simulink model "BD_PAR_AUTO_base_model"  (Simulink 10.3)
settings: Solver=ode1  StartTime=0.0  StopTime=max(cyc_mph(:,1))  FixedStep=1  MaxStep=1  RelTol=1e-3  AbsTol=1e-3
undefined symbols (not defined in the file): acc_dcdc_eff, acc_elec_eff, acc_elec_pwr, acc_mech_eff, acc_mech_pwr, acc_mech_trq, air_cp, amb_tmp, cs_charge_deplete_bool, cs_charge_trq, cs_electric_decel_spd, cs_electric_launch_spd_hi, cs_electric_launch_spd_lo, cs_hi_soc, cs_lo_soc, cs_min_trq_frac, cs_off_trq_frac, cyc_avg_time, cyc_cargo_mass, cyc_elevation_init, cyc_filter_bool, cyc_grade, cyc_mph, enable_sim_stop_distance, enable_sim_stop_max_spd, enable_sim_stop_speed, enable_sim_stop_time, enable_stop, enable_stop_fc, ess_cap_scale, ess_coulombic_eff, ess_init_soc, ess_max_ah_cap, ess_max_volts, ess_min_volts, ess_mod_airflow, ess_mod_cp, ess_mod_init_tmp, ess_module_mass, ess_module_num, ess_on, ess_r_chg, ess_r_dis, ess_res_scale_coef, ess_res_scale_fun, ess_set_tmp, ess_soc, ess_th_calc, ess_th_res_off, ess_th_res_on, ess_tmp, ess_voc, ex_calc, ex_cat_co_frac, ex_cat_ext_cp, ex_cat_ext_emisv, ex_cat_ext_init_tmp, ex_cat_ext_mass, ex_cat_ext_sarea, ex_cat_hc_frac ... (+168)
(part 14 of 15)

== system BD_PAR_AUTO_base_model/electric acc loads <acc>/Electrical Accessory Loads v2 <acc>/backward model/electrical accessories (W)/Electrical Accessories: Time Variable/Elec Aux Loads 14V Pwr/RearHVAC/Subsystem/Subsystem1/ToggleTimes ==
  Constant : Constant  Value=ToggleTimes  VectorParams1D=off
  Out1 : Outport
  wires:
  Constant/1 -> Out1/1

== system BD_PAR_AUTO_base_model/electric acc loads <acc>/Electrical Accessory Loads v2 <acc>/backward model/electrical accessories (W)/Electrical Accessories: Time Variable/Elec Aux Loads 14V Pwr/RearHVAC/Subsystem/Subsystem1/Triggered Subsystem1 ==
  In1 : Inport
  Enable : EnablePort
  Constant1 : Constant
  Constant2 : Constant  Value=0
  Constant3 : Constant  Value=0
  Relational Operator : RelationalOperator  Operator===  RndMeth=Nearest  InputSameDT=on
  Switch : Switch  Threshold=.5
  Out1 : Outport  InitialOutput=InitialOn
  wires:
  Switch/1 -> Out1/1
  Constant3/1 -> Switch/3
  Constant1/1 -> Switch/1
  Relational Operator/1 -> Switch/2
  Constant2/1 -> Relational Operator/2
  In1/1 -> Relational Operator/1

== system BD_PAR_AUTO_base_model/electric acc loads <acc>/Electrical Accessory Loads v2 <acc>/backward model/electrical accessories (W)/Electrical Accessories: Time Variable/Elec Aux Loads 14V Pwr/RearWipers/Subsystem/Subsystem/DurationOn1 ==
  Constant : Constant  Value=DurationOn
  Out1 : Outport
  wires:
  Constant/1 -> Out1/1

== system BD_PAR_AUTO_base_model/electric acc loads <acc>/Electrical Accessory Loads v2 <acc>/backward model/electrical accessories (W)/Electrical Accessories: Time Variable/Elec Aux Loads 14V Pwr/RearWipers/Subsystem/Subsystem/Period1 ==
  Constant : Constant  Value=Period
  Out1 : Outport
  wires:
  Constant/1 -> Out1/1

== system BD_PAR_AUTO_base_model/electric acc loads <acc>/Electrical Accessory Loads v2 <acc>/backward model/electrical accessories (W)/Electrical Accessories: Time Variable/Elec Aux Loads 14V Pwr/RearWipers/Subsystem/Subsystem/StartTime1 ==
  Constant : Constant  Value=StartTime
  Out1 : Outport
  wires:
  Constant/1 -> Out1/1

== system BD_PAR_AUTO_base_model/electric acc loads <acc>/Electrical Accessory Loads v2 <acc>/backward model/electrical accessories (W)/Electrical Accessories: Time Variable/Elec Aux Loads 14V Pwr/RearWipers/Subsystem/Subsystem/StartTime3 ==
  Constant : Constant  Value=StartTime
  Out1 : Outport
  wires:
  Constant/1 -> Out1/1

== system BD_PAR_AUTO_base_model/electric acc loads <acc>/Electrical Accessory Loads v2 <acc>/backward model/electrical accessories (W)/Electrical Accessories: Time Variable/Elec Aux Loads 14V Pwr/RearWipers/Subsystem/Subsystem/Triggered Subsystem2 ==
  time : Inport
  Trigger : TriggerPort  VariantControl=(inherit)
  last trig on time : Outport  InitialOutput=StartTime
  wires:
  time/1 -> last trig on time/1

== system BD_PAR_AUTO_base_model/electric acc loads <acc>/Electrical Accessory Loads v2 <acc>/backward model/electrical accessories (W)/Electrical Accessories: Time Variable/Elec Aux Loads 14V Pwr/RearWipers/Subsystem/Subsystem1/ToggleTimes ==
  Constant : Constant  Value=ToggleTimes  VectorParams1D=off
  Out1 : Outport
  wires:
  Constant/1 -> Out1/1

== system BD_PAR_AUTO_base_model/electric acc loads <acc>/Electrical Accessory Loads v2 <acc>/backward model/electrical accessories (W)/Electrical Accessories: Time Variable/Elec Aux Loads 14V Pwr/RearWipers/Subsystem/Subsystem1/Triggered Subsystem1 ==
  In1 : Inport
  Enable : EnablePort
  Constant1 : Constant
  Constant2 : Constant  Value=0
  Constant3 : Constant  Value=0
  Relational Operator : RelationalOperator  Operator===  RndMeth=Nearest  InputSameDT=on
  Switch : Switch  Threshold=.5
  Out1 : Outport  InitialOutput=InitialOn
  wires:
  Switch/1 -> Out1/1
  Constant3/1 -> Switch/3
  Constant1/1 -> Switch/1
  Relational Operator/1 -> Switch/2
  Constant2/1 -> Relational Operator/2
  In1/1 -> Relational Operator/1

== system BD_PAR_AUTO_base_model/electric acc loads <acc>/Electrical Accessory Loads v2 <acc>/backward model/electrical accessories (W)/Electrical Accessories: Time Variable/Elec Aux Loads 14V Pwr/Starter/Starter/Subsystem/Last Engine On Time ==
  In1 : Inport
  Trigger : TriggerPort  VariantControl=(inherit)
  Out1 : Outport  InitialOutput=-100
  wires:
  In1/1 -> Out1/1

== system BD_PAR_AUTO_base_model/electric acc loads <acc>/Electrical Accessory Loads v2 <acc>/backward model/electrical accessories (W)/Electrical Accessories: Time Variable/Elec Aux Loads 14V Pwr/TurnSignals/Subsystem/Subsystem/DurationOn1 ==
  Constant : Constant  Value=DurationOn
  Out1 : Outport
  wires:
  Constant/1 -> Out1/1

== system BD_PAR_AUTO_base_model/electric acc loads <acc>/Electrical Accessory Loads v2 <acc>/backward model/electrical accessories (W)/Electrical Accessories: Time Variable/Elec Aux Loads 14V Pwr/TurnSignals/Subsystem/Subsystem/Period1 ==
  Constant : Constant  Value=Period
  Out1 : Outport
  wires:
  Constant/1 -> Out1/1

== system BD_PAR_AUTO_base_model/electric acc loads <acc>/Electrical Accessory Loads v2 <acc>/backward model/electrical accessories (W)/Electrical Accessories: Time Variable/Elec Aux Loads 14V Pwr/TurnSignals/Subsystem/Subsystem/StartTime1 ==
  Constant : Constant  Value=StartTime
  Out1 : Outport
  wires:
  Constant/1 -> Out1/1

== system BD_PAR_AUTO_base_model/electric acc loads <acc>/Electrical Accessory Loads v2 <acc>/backward model/electrical accessories (W)/Electrical Accessories: Time Variable/Elec Aux Loads 14V Pwr/TurnSignals/Subsystem/Subsystem/StartTime3 ==
  Constant : Constant  Value=StartTime
  Out1 : Outport
  wires:
  Constant/1 -> Out1/1

== system BD_PAR_AUTO_base_model/electric acc loads <acc>/Electrical Accessory Loads v2 <acc>/backward model/electrical accessories (W)/Electrical Accessories: Time Variable/Elec Aux Loads 14V Pwr/TurnSignals/Subsystem/Subsystem/Triggered Subsystem2 ==
  time : Inport
  Trigger : TriggerPort  VariantControl=(inherit)
  last trig on time : Outport  InitialOutput=StartTime
  wires:
  time/1 -> last trig on time/1

== system BD_PAR_AUTO_base_model/electric acc loads <acc>/Electrical Accessory Loads v2 <acc>/backward model/electrical accessories (W)/Electrical Accessories: Time Variable/Elec Aux Loads 14V Pwr/TurnSignals/Subsystem/Subsystem1/ToggleTimes ==
  Constant : Constant  Value=ToggleTimes  VectorParams1D=off
  Out1 : Outport
  wires:
  Constant/1 -> Out1/1

== system BD_PAR_AUTO_base_model/electric acc loads <acc>/Electrical Accessory Loads v2 <acc>/backward model/electrical accessories (W)/Electrical Accessories: Time Variable/Elec Aux Loads 14V Pwr/TurnSignals/Subsystem/Subsystem1/Triggered Subsystem1 ==
  In1 : Inport
  Enable : EnablePort
  Constant1 : Constant
  Constant2 : Constant  Value=0
  Constant3 : Constant  Value=0
  Relational Operator : RelationalOperator  Operator===  RndMeth=Nearest  InputSameDT=on
  Switch : Switch  Threshold=.5
  Out1 : Outport  InitialOutput=InitialOn
  wires:
  Switch/1 -> Out1/1
  Constant3/1 -> Switch/3
  Constant1/1 -> Switch/1
  Relational Operator/1 -> Switch/2
  Constant2/1 -> Relational Operator/2
  In1/1 -> Relational Operator/1

== system BD_PAR_AUTO_base_model/electric acc loads <acc>/Electrical Accessory Loads v2 <acc>/backward model/electrical accessories (W)/Electrical Accessories: Time Variable/Elec Aux Loads HiV Pwr/CurrentLoad1/Subsystem/Subsystem/DurationOn1 ==
  Constant : Constant  Value=DurationOn
  Out1 : Outport
  wires:
  Constant/1 -> Out1/1

== system BD_PAR_AUTO_base_model/electric acc loads <acc>/Electrical Accessory Loads v2 <acc>/backward model/electrical accessories (W)/Electrical Accessories: Time Variable/Elec Aux Loads HiV Pwr/CurrentLoad1/Subsystem/Subsystem/Period1 ==
  Constant : Constant  Value=Period
  Out1 : Outport
  wires:
  Constant/1 -> Out1/1

== system BD_PAR_AUTO_base_model/electric acc loads <acc>/Electrical Accessory Loads v2 <acc>/backward model/electrical accessories (W)/Electrical Accessories: Time Variable/Elec Aux Loads HiV Pwr/CurrentLoad1/Subsystem/Subsystem/StartTime1 ==
  Constant : Constant  Value=StartTime
  Out1 : Outport
  wires:
  Constant/1 -> Out1/1

== system BD_PAR_AUTO_base_model/electric acc loads <acc>/Electrical Accessory Loads v2 <acc>/backward model/electrical accessories (W)/Electrical Accessories: Time Variable/Elec Aux Loads HiV Pwr/CurrentLoad1/Subsystem/Subsystem/StartTime3 ==
  Constant : Constant  Value=StartTime
  Out1 : Outport
  wires:
  Constant/1 -> Out1/1

== system BD_PAR_AUTO_base_model/electric acc loads <acc>/Electrical Accessory Loads v2 <acc>/backward model/electrical accessories (W)/Electrical Accessories: Time Variable/Elec Aux Loads HiV Pwr/CurrentLoad1/Subsystem/Subsystem/Triggered Subsystem2 ==
  time : Inport
  Trigger : TriggerPort  VariantControl=(inherit)
  last trig on time : Outport  InitialOutput=StartTime
  wires:
  time/1 -> last trig on time/1

== system BD_PAR_AUTO_base_model/electric acc loads <acc>/Electrical Accessory Loads v2 <acc>/backward model/electrical accessories (W)/Electrical Accessories: Time Variable/Elec Aux Loads HiV Pwr/CurrentLoad1/Subsystem/Subsystem1/ToggleTimes ==
  Constant : Constant  Value=ToggleTimes  VectorParams1D=off
  Out1 : Outport
  wires:
  Constant/1 -> Out1/1

== system BD_PAR_AUTO_base_model/electric acc loads <acc>/Electrical Accessory Loads v2 <acc>/backward model/electrical accessories (W)/Electrical Accessories: Time Variable/Elec Aux Loads HiV Pwr/CurrentLoad1/Subsystem/Subsystem1/Triggered Subsystem1 ==
  In1 : Inport
  Enable : EnablePort
  Constant1 : Constant
  Constant2 : Constant  Value=0
  Constant3 : Constant  Value=0
  Relational Operator : RelationalOperator  Operator===  RndMeth=Nearest  InputSameDT=on
  Switch : Switch  Threshold=.5
  Out1 : Outport  InitialOutput=InitialOn
  wires:
  Switch/1 -> Out1/1
  Constant3/1 -> Switch/3
  Constant1/1 -> Switch/1
  Relational Operator/1 -> Switch/2
  Constant2/1 -> Relational Operator/2
  In1/1 -> Relational Operator/1

== system BD_PAR_AUTO_base_model/electric acc loads <acc>/Electrical Accessory Loads v2 <acc>/backward model/electrical accessories (W)/Electrical Accessories: Time Variable/Elec Aux Loads HiV Pwr/PowerLoad1/Subsystem/Subsystem/DurationOn1 ==
  Constant : Constant  Value=DurationOn
  Out1 : Outport
  wires:
  Constant/1 -> Out1/1

== system BD_PAR_AUTO_base_model/electric acc loads <acc>/Electrical Accessory Loads v2 <acc>/backward model/electrical accessories (W)/Electrical Accessories: Time Variable/Elec Aux Loads HiV Pwr/PowerLoad1/Subsystem/Subsystem/Period1 ==
  Constant : Constant  Value=Period
  Out1 : Outport
  wires:
  Constant/1 -> Out1/1

== system BD_PAR_AUTO_base_model/electric acc loads <acc>/Electrical Accessory Loads v2 <acc>/backward model/electrical accessories (W)/Electrical Accessories: Time Variable/Elec Aux Loads HiV Pwr/PowerLoad1/Subsystem/Subsystem/StartTime1 ==
  Constant : Constant  Value=StartTime
  Out1 : Outport
  wires:
  Constant/1 -> Out1/1

== system BD_PAR_AUTO_base_model/electric acc loads <acc>/Electrical Accessory Loads v2 <acc>/backward model/electrical accessories (W)/Electrical Accessories: Time Variable/Elec Aux Loads HiV Pwr/PowerLoad1/Subsystem/Subsystem/StartTime3 ==
  Constant : Constant  Value=StartTime
  Out1 : Outport
  wires:
  Constant/1 -> Out1/1

== system BD_PAR_AUTO_base_model/electric acc loads <acc>/Electrical Accessory Loads v2 <acc>/backward model/electrical accessories (W)/Electrical Accessories: Time Variable/Elec Aux Loads HiV Pwr/PowerLoad1/Subsystem/Subsystem/Triggered Subsystem2 ==
  time : Inport
  Trigger : TriggerPort  VariantControl=(inherit)
  last trig on time : Outport  InitialOutput=StartTime
  wires:
  time/1 -> last trig on time/1

== system BD_PAR_AUTO_base_model/electric acc loads <acc>/Electrical Accessory Loads v2 <acc>/backward model/electrical accessories (W)/Electrical Accessories: Time Variable/Elec Aux Loads HiV Pwr/PowerLoad1/Subsystem/Subsystem1/ToggleTimes ==
  Constant : Constant  Value=ToggleTimes  VectorParams1D=off
  Out1 : Outport
  wires:
  Constant/1 -> Out1/1

== system BD_PAR_AUTO_base_model/electric acc loads <acc>/Electrical Accessory Loads v2 <acc>/backward model/electrical accessories (W)/Electrical Accessories: Time Variable/Elec Aux Loads HiV Pwr/PowerLoad1/Subsystem/Subsystem1/Triggered Subsystem1 ==
  In1 : Inport
  Enable : EnablePort
  Constant1 : Constant
  Constant2 : Constant  Value=0
  Constant3 : Constant  Value=0
  Relational Operator : RelationalOperator  Operator===  RndMeth=Nearest  InputSameDT=on
  Switch : Switch  Threshold=.5
  Out1 : Outport  InitialOutput=InitialOn
  wires:
  Switch/1 -> Out1/1
  Constant3/1 -> Switch/3
  Constant1/1 -> Switch/1
  Relational Operator/1 -> Switch/2
  Constant2/1 -> Relational Operator/2
  In1/1 -> Relational Operator/1

== system BD_PAR_AUTO_base_model/electric acc loads <acc>/Electrical Accessory Loads v2 <acc>/backward model/electrical accessories (W)/Electrical Accessories: Time Variable/Elec Aux Loads HiV Pwr/PowerLoad2/Subsystem/Subsystem/DurationOn1 ==
  Constant : Constant  Value=DurationOn
  Out1 : Outport
  wires:
  Constant/1 -> Out1/1

== system BD_PAR_AUTO_base_model/electric acc loads <acc>/Electrical Accessory Loads v2 <acc>/backward model/electrical accessories (W)/Electrical Accessories: Time Variable/Elec Aux Loads HiV Pwr/PowerLoad2/Subsystem/Subsystem/Period1 ==
  Constant : Constant  Value=Period
  Out1 : Outport
  wires:
  Constant/1 -> Out1/1

== system BD_PAR_AUTO_base_model/electric acc loads <acc>/Electrical Accessory Loads v2 <acc>/backward model/electrical accessories (W)/Electrical Accessories: Time Variable/Elec Aux Loads HiV Pwr/PowerLoad2/Subsystem/Subsystem/StartTime1 ==
  Constant : Constant  Value=StartTime
  Out1 : Outport
  wires:
  Constant/1 -> Out1/1

== system BD_PAR_AUTO_base_model/electric acc loads <acc>/Electrical Accessory Loads v2 <acc>/backward model/electrical accessories (W)/Electrical Accessories: Time Variable/Elec Aux Loads HiV Pwr/PowerLoad2/Subsystem/Subsystem/StartTime3 ==
  Constant : Constant  Value=StartTime
  Out1 : Outport
  wires:
  Constant/1 -> Out1/1

== system BD_PAR_AUTO_base_model/electric acc loads <acc>/Electrical Accessory Loads v2 <acc>/backward model/electrical accessories (W)/Electrical Accessories: Time Variable/Elec Aux Loads HiV Pwr/PowerLoad2/Subsystem/Subsystem/Triggered Subsystem2 ==
  time : Inport
  Trigger : TriggerPort  VariantControl=(inherit)
  last trig on time : Outport  InitialOutput=StartTime
  wires:
  time/1 -> last trig on time/1

== system BD_PAR_AUTO_base_model/electric acc loads <acc>/Electrical Accessory Loads v2 <acc>/backward model/electrical accessories (W)/Electrical Accessories: Time Variable/Elec Aux Loads HiV Pwr/PowerLoad2/Subsystem/Subsystem1/ToggleTimes ==
  Constant : Constant  Value=ToggleTimes  VectorParams1D=off
  Out1 : Outport
  wires:
  Constant/1 -> Out1/1

== system BD_PAR_AUTO_base_model/electric acc loads <acc>/Electrical Accessory Loads v2 <acc>/backward model/electrical accessories (W)/Electrical Accessories: Time Variable/Elec Aux Loads HiV Pwr/PowerLoad2/Subsystem/Subsystem1/Triggered Subsystem1 ==
  In1 : Inport
  Enable : EnablePort
  Constant1 : Constant
  Constant2 : Constant  Value=0
  Constant3 : Constant  Value=0
  Relational Operator : RelationalOperator  Operator===  RndMeth=Nearest  InputSameDT=on
  Switch : Switch  Threshold=.5
  Out1 : Outport  InitialOutput=InitialOn
  wires:
  Switch/1 -> Out1/1
  Constant3/1 -> Switch/3
  Constant1/1 -> Switch/1
  Relational Operator/1 -> Switch/2
  Constant2/1 -> Relational Operator/2
  In1/1 -> Relational Operator/1

== system BD_PAR_AUTO_base_model/electric acc loads <acc>/Electrical Accessory Loads v2 <acc>/backward model/electrical accessories (W)/Electrical Accessories: Time Variable/Elec Aux Loads HiV Pwr/PowerLoad3/Subsystem/Subsystem/DurationOn1 ==
  Constant : Constant  Value=DurationOn
  Out1 : Outport
  wires:
  Constant/1 -> Out1/1

== system BD_PAR_AUTO_base_model/electric acc loads <acc>/Electrical Accessory Loads v2 <acc>/backward model/electrical accessories (W)/Electrical Accessories: Time Variable/Elec Aux Loads HiV Pwr/PowerLoad3/Subsystem/Subsystem/Period1 ==
  Constant : Constant  Value=Period
  Out1 : Outport
  wires:
  Constant/1 -> Out1/1

== system BD_PAR_AUTO_base_model/electric acc loads <acc>/Electrical Accessory Loads v2 <acc>/backward model/electrical accessories (W)/Electrical Accessories: Time Variable/Elec Aux Loads HiV Pwr/PowerLoad3/Subsystem/Subsystem/StartTime1 ==
  Constant : Constant  Value=StartTime
  Out1 : Outport
  wires:
  Constant/1 -> Out1/1

== system BD_PAR_AUTO_base_model/electric acc loads <acc>/Electrical Accessory Loads v2 <acc>/backward model/electrical accessories (W)/Electrical Accessories: Time Variable/Elec Aux Loads HiV Pwr/PowerLoad3/Subsystem/Subsystem/StartTime3 ==
  Constant : Constant  Value=StartTime
  Out1 : Outport
  wires:
  Constant/1 -> Out1/1

== system BD_PAR_AUTO_base_model/electric acc loads <acc>/Electrical Accessory Loads v2 <acc>/backward model/electrical accessories (W)/Electrical Accessories: Time Variable/Elec Aux Loads HiV Pwr/PowerLoad3/Subsystem/Subsystem/Triggered Subsystem2 ==
  time : Inport
  Trigger : TriggerPort  VariantControl=(inherit)
  last trig on time : Outport  InitialOutput=StartTime
  wires:
  time/1 -> last trig on time/1

== system BD_PAR_AUTO_base_model/electric acc loads <acc>/Electrical Accessory Loads v2 <acc>/backward model/electrical accessories (W)/Electrical Accessories: Time Variable/Elec Aux Loads HiV Pwr/PowerLoad3/Subsystem/Subsystem1/ToggleTimes ==
  Constant : Constant  Value=ToggleTimes  VectorParams1D=off
  Out1 : Outport
  wires:
  Constant/1 -> Out1/1

== system BD_PAR_AUTO_base_model/electric acc loads <acc>/Electrical Accessory Loads v2 <acc>/backward model/electrical accessories (W)/Electrical Accessories: Time Variable/Elec Aux Loads HiV Pwr/PowerLoad3/Subsystem/Subsystem1/Triggered Subsystem1 ==
  In1 : Inport
  Enable : EnablePort
  Constant1 : Constant
  Constant2 : Constant  Value=0
  Constant3 : Constant  Value=0
  Relational Operator : RelationalOperator  Operator===  RndMeth=Nearest  InputSameDT=on
  Switch : Switch  Threshold=.5
  Out1 : Outport  InitialOutput=InitialOn
  wires:
  Switch/1 -> Out1/1
  Constant3/1 -> Switch/3
  Constant1/1 -> Switch/1
  Relational Operator/1 -> Switch/2
  Constant2/1 -> Relational Operator/2
  In1/1 -> Relational Operator/1

== system BD_PAR_AUTO_base_model/electric acc loads <acc>/Electrical Accessory Loads v2 <acc>/backward model/electrical accessories (W)/Electrical Accessories: Time Variable/Elec Aux Loads HiV Pwr/SpeedLoad1/Subsystem/Subsystem/DurationOn1 ==
  Constant : Constant  Value=DurationOn
  Out1 : Outport
  wires:
  Constant/1 -> Out1/1

== system BD_PAR_AUTO_base_model/electric acc loads <acc>/Electrical Accessory Loads v2 <acc>/backward model/electrical accessories (W)/Electrical Accessories: Time Variable/Elec Aux Loads HiV Pwr/SpeedLoad1/Subsystem/Subsystem/Period1 ==
  Constant : Constant  Value=Period
  Out1 : Outport
  wires:
  Constant/1 -> Out1/1

== system BD_PAR_AUTO_base_model/electric acc loads <acc>/Electrical Accessory Loads v2 <acc>/backward model/electrical accessories (W)/Electrical Accessories: Time Variable/Elec Aux Loads HiV Pwr/SpeedLoad1/Subsystem/Subsystem/StartTime1 ==
  Constant : Constant  Value=StartTime
  Out1 : Outport
  wires:
  Constant/1 -> Out1/1

== system BD_PAR_AUTO_base_model/electric acc loads <acc>/Electrical Accessory Loads v2 <acc>/backward model/electrical accessories (W)/Electrical Accessories: Time Variable/Elec Aux Loads HiV Pwr/SpeedLoad1/Subsystem/Subsystem/StartTime3 ==
  Constant : Constant  Value=StartTime
  Out1 : Outport
  wires:
  Constant/1 -> Out1/1

== system BD_PAR_AUTO_base_model/electric acc loads <acc>/Electrical Accessory Loads v2 <acc>/backward model/electrical accessories (W)/Electrical Accessories: Time Variable/Elec Aux Loads HiV Pwr/SpeedLoad1/Subsystem/Subsystem/Triggered Subsystem2 ==
  time : Inport
  Trigger : TriggerPort  VariantControl=(inherit)
  last trig on time : Outport  InitialOutput=StartTime
  wires:
  time/1 -> last trig on time/1

== system BD_PAR_AUTO_base_model/electric acc loads <acc>/Electrical Accessory Loads v2 <acc>/backward model/electrical accessories (W)/Electrical Accessories: Time Variable/Elec Aux Loads HiV Pwr/SpeedLoad1/Subsystem/Subsystem1/ToggleTimes ==
  Constant : Constant  Value=ToggleTimes  VectorParams1D=off
  Out1 : Outport
  wires:
  Constant/1 -> Out1/1

== system BD_PAR_AUTO_base_model/electric acc loads <acc>/Electrical Accessory Loads v2 <acc>/backward model/electrical accessories (W)/Electrical Accessories: Time Variable/Elec Aux Loads HiV Pwr/SpeedLoad1/Subsystem/Subsystem1/Triggered Subsystem1 ==
  In1 : Inport
  Enable : EnablePort
  Constant1 : Constant
  Constant2 : Constant  Value=0
  Constant3 : Constant  Value=0
  Relational Operator : RelationalOperator  Operator===  RndMeth=Nearest  InputSameDT=on
  Switch : Switch  Threshold=.5
  Out1 : Outport  InitialOutput=InitialOn
  wires:
  Switch/1 -> Out1/1
  Constant3/1 -> Switch/3
  Constant1/1 -> Switch/1
  Relational Operator/1 -> Switch/2
  Constant2/1 -> Relational Operator/2
  In1/1 -> Relational Operator/1

== system BD_PAR_AUTO_base_model/electric acc loads <acc>/Electrical Accessory Loads v2 <acc>/backward model/electrical accessories (W)/Electrical Accessories: Time Variable/Elec Aux Loads HiV Pwr/Starter/Starter/Subsystem/Last Engine On Time ==
  In1 : Inport
  Trigger : TriggerPort  VariantControl=(inherit)
  Out1 : Outport  InitialOutput=-100
  wires:
  In1/1 -> Out1/1

== system BD_PAR_AUTO_base_model/mechanical accessory loads <acc>/Mechanical Accessory Loads v2 <acc>/backward model/mechanical accessories (Nm)/Mechanical Accessories: Const Mech Var Elect/Elec Aux Loads 14V Pwr/ExternalLights/Subsystem/Subsystem/DurationOn1 ==
  Constant : Constant  Value=DurationOn
  Out1 : Outport
  wires:
  Constant/1 -> Out1/1

== system BD_PAR_AUTO_base_model/mechanical accessory loads <acc>/Mechanical Accessory Loads v2 <acc>/backward model/mechanical accessories (Nm)/Mechanical Accessories: Const Mech Var Elect/Elec Aux Loads 14V Pwr/ExternalLights/Subsystem/Subsystem/Period1 ==
  Constant : Constant  Value=Period
  Out1 : Outport
  wires:
  Constant/1 -> Out1/1

== system BD_PAR_AUTO_base_model/mechanical accessory loads <acc>/Mechanical Accessory Loads v2 <acc>/backward model/mechanical accessories (Nm)/Mechanical Accessories: Const Mech Var Elect/Elec Aux Loads 14V Pwr/ExternalLights/Subsystem/Subsystem/StartTime1 ==
  Constant : Constant  Value=StartTime
  Out1 : Outport
  wires:
  Constant/1 -> Out1/1

== system BD_PAR_AUTO_base_model/mechanical accessory loads <acc>/Mechanical Accessory Loads v2 <acc>/backward model/mechanical accessories (Nm)/Mechanical Accessories: Const Mech Var Elect/Elec Aux Loads 14V Pwr/ExternalLights/Subsystem/Subsystem/StartTime3 ==
  Constant : Constant  Value=StartTime
  Out1 : Outport
  wires:
  Constant/1 -> Out1/1

== system BD_PAR_AUTO_base_model/mechanical accessory loads <acc>/Mechanical Accessory Loads v2 <acc>/backward model/mechanical accessories (Nm)/Mechanical Accessories: Const Mech Var Elect/Elec Aux Loads 14V Pwr/ExternalLights/Subsystem/Subsystem/Triggered Subsystem2 ==
  time : Inport
  Trigger : TriggerPort  VariantControl=(inherit)
  last trig on time : Outport  InitialOutput=StartTime
  wires:
  time/1 -> last trig on time/1

== system BD_PAR_AUTO_base_model/mechanical accessory loads <acc>/Mechanical Accessory Loads v2 <acc>/backward model/mechanical accessories (Nm)/Mechanical Accessories: Const Mech Var Elect/Elec Aux Loads 14V Pwr/ExternalLights/Subsystem/Subsystem1/ToggleTimes ==
  Constant : Constant  Value=ToggleTimes  VectorParams1D=off
  Out1 : Outport
  wires:
  Constant/1 -> Out1/1

== system BD_PAR_AUTO_base_model/mechanical accessory loads <acc>/Mechanical Accessory Loads v2 <acc>/backward model/mechanical accessories (Nm)/Mechanical Accessories: Const Mech Var Elect/Elec Aux Loads 14V Pwr/ExternalLights/Subsystem/Subsystem1/Triggered Subsystem1 ==
  In1 : Inport
  Enable : EnablePort
  Constant1 : Constant
  Constant2 : Constant  Value=0
  Constant3 : Constant  Value=0
  Relational Operator : RelationalOperator  Operator===  RndMeth=Nearest  InputSameDT=on
  Switch : Switch  Threshold=.5
  Out1 : Outport  InitialOutput=InitialOn
  wires:
  Switch/1 -> Out1/1
  Constant3/1 -> Switch/3
  Constant1/1 -> Switch/1
  Relational Operator/1 -> Switch/2
  Constant2/1 -> Relational Operator/2
  In1/1 -> Relational Operator/1

== system BD_PAR_AUTO_base_model/mechanical accessory loads <acc>/Mechanical Accessory Loads v2 <acc>/backward model/mechanical accessories (Nm)/Mechanical Accessories: Const Mech Var Elect/Elec Aux Loads 14V Pwr/FrontHVAC/Subsystem/Subsystem/DurationOn1 ==
  Constant : Constant  Value=DurationOn
  Out1 : Outport
  wires:
  Constant/1 -> Out1/1

== system BD_PAR_AUTO_base_model/mechanical accessory loads <acc>/Mechanical Accessory Loads v2 <acc>/backward model/mechanical accessories (Nm)/Mechanical Accessories: Const Mech Var Elect/Elec Aux Loads 14V Pwr/FrontHVAC/Subsystem/Subsystem/Period1 ==
  Constant : Constant  Value=Period
  Out1 : Outport
  wires:
  Constant/1 -> Out1/1

== system BD_PAR_AUTO_base_model/mechanical accessory loads <acc>/Mechanical Accessory Loads v2 <acc>/backward model/mechanical accessories (Nm)/Mechanical Accessories: Const Mech Var Elect/Elec Aux Loads 14V Pwr/FrontHVAC/Subsystem/Subsystem/StartTime1 ==
  Constant : Constant  Value=StartTime
  Out1 : Outport
  wires:
  Constant/1 -> Out1/1

== system BD_PAR_AUTO_base_model/mechanical accessory loads <acc>/Mechanical Accessory Loads v2 <acc>/backward model/mechanical accessories (Nm)/Mechanical Accessories: Const Mech Var Elect/Elec Aux Loads 14V Pwr/FrontHVAC/Subsystem/Subsystem/StartTime3 ==
  Constant : Constant  Value=StartTime
  Out1 : Outport
  wires:
  Constant/1 -> Out1/1

== system BD_PAR_AUTO_base_model/mechanical accessory loads <acc>/Mechanical Accessory Loads v2 <acc>/backward model/mechanical accessories (Nm)/Mechanical Accessories: Const Mech Var Elect/Elec Aux Loads 14V Pwr/FrontHVAC/Subsystem/Subsystem/Triggered Subsystem2 ==
  time : Inport
  Trigger : TriggerPort  VariantControl=(inherit)
  last trig on time : Outport  InitialOutput=StartTime
  wires:
  time/1 -> last trig on time/1

== system BD_PAR_AUTO_base_model/mechanical accessory loads <acc>/Mechanical Accessory Loads v2 <acc>/backward model/mechanical accessories (Nm)/Mechanical Accessories: Const Mech Var Elect/Elec Aux Loads 14V Pwr/FrontHVAC/Subsystem/Subsystem1/ToggleTimes ==
  Constant : Constant  Value=ToggleTimes  VectorParams1D=off
  Out1 : Outport
  wires:
  Constant/1 -> Out1/1

== system BD_PAR_AUTO_base_model/mechanical accessory loads <acc>/Mechanical Accessory Loads v2 <acc>/backward model/mechanical accessories (Nm)/Mechanical Accessories: Const Mech Var Elect/Elec Aux Loads 14V Pwr/FrontHVAC/Subsystem/Subsystem1/Triggered Subsystem1 ==
  In1 : Inport
  Enable : EnablePort
  Constant1 : Constant
  Constant2 : Constant  Value=0
  Constant3 : Constant  Value=0
  Relational Operator : RelationalOperator  Operator===  RndMeth=Nearest  InputSameDT=on
  Switch : Switch  Threshold=.5
  Out1 : Outport  InitialOutput=InitialOn
  wires:
  Switch/1 -> Out1/1
  Constant3/1 -> Switch/3
  Constant1/1 -> Switch/1
  Relational Operator/1 -> Switch/2
  Constant2/1 -> Relational Operator/2
  In1/1 -> Relational Operator/1

== system BD_PAR_AUTO_base_model/mechanical accessory loads <acc>/Mechanical Accessory Loads v2 <acc>/backward model/mechanical accessories (Nm)/Mechanical Accessories: Const Mech Var Elect/Elec Aux Loads 14V Pwr/FrontWipers/Subsystem/Subsystem/DurationOn1 ==
  Constant : Constant  Value=DurationOn
  Out1 : Outport
  wires:
  Constant/1 -> Out1/1

== system BD_PAR_AUTO_base_model/mechanical accessory loads <acc>/Mechanical Accessory Loads v2 <acc>/backward model/mechanical accessories (Nm)/Mechanical Accessories: Const Mech Var Elect/Elec Aux Loads 14V Pwr/FrontWipers/Subsystem/Subsystem/Period1 ==
  Constant : Constant  Value=Period
  Out1 : Outport
  wires:
  Constant/1 -> Out1/1

== system BD_PAR_AUTO_base_model/mechanical accessory loads <acc>/Mechanical Accessory Loads v2 <acc>/backward model/mechanical accessories (Nm)/Mechanical Accessories: Const Mech Var Elect/Elec Aux Loads 14V Pwr/FrontWipers/Subsystem/Subsystem/StartTime1 ==
  Constant : Constant  Value=StartTime
  Out1 : Outport
  wires:
  Constant/1 -> Out1/1

== system BD_PAR_AUTO_base_model/mechanical accessory loads <acc>/Mechanical Accessory Loads v2 <acc>/backward model/mechanical accessories (Nm)/Mechanical Accessories: Const Mech Var Elect/Elec Aux Loads 14V Pwr/FrontWipers/Subsystem/Subsystem/StartTime3 ==
  Constant : Constant  Value=StartTime
  Out1 : Outport
  wires:
  Constant/1 -> Out1/1

== system BD_PAR_AUTO_base_model/mechanical accessory loads <acc>/Mechanical Accessory Loads v2 <acc>/backward model/mechanical accessories (Nm)/Mechanical Accessories: Const Mech Var Elect/Elec Aux Loads 14V Pwr/FrontWipers/Subsystem/Subsystem/Triggered Subsystem2 ==
  time : Inport
  Trigger : TriggerPort  VariantControl=(inherit)
  last trig on time : Outport  InitialOutput=StartTime
  wires:
  time/1 -> last trig on time/1

== system BD_PAR_AUTO_base_model/mechanical accessory loads <acc>/Mechanical Accessory Loads v2 <acc>/backward model/mechanical accessories (Nm)/Mechanical Accessories: Const Mech Var Elect/Elec Aux Loads 14V Pwr/FrontWipers/Subsystem/Subsystem1/ToggleTimes ==
  Constant : Constant  Value=ToggleTimes  VectorParams1D=off
  Out1 : Outport
  wires:
  Constant/1 -> Out1/1

== system BD_PAR_AUTO_base_model/mechanical accessory loads <acc>/Mechanical Accessory Loads v2 <acc>/backward model/mechanical accessories (Nm)/Mechanical Accessories: Const Mech Var Elect/Elec Aux Loads 14V Pwr/FrontWipers/Subsystem/Subsystem1/Triggered Subsystem1 ==
  In1 : Inport
  Enable : EnablePort
  Constant1 : Constant
  Constant2 : Constant  Value=0
  Constant3 : Constant  Value=0
  Relational Operator : RelationalOperator  Operator===  RndMeth=Nearest  InputSameDT=on
  Switch : Switch  Threshold=.5
  Out1 : Outport  InitialOutput=InitialOn
  wires:
  Switch/1 -> Out1/1
  Constant3/1 -> Switch/3
  Constant1/1 -> Switch/1
  Relational Operator/1 -> Switch/2
  Constant2/1 -> Relational Operator/2
  In1/1 -> Relational Operator/1

== system BD_PAR_AUTO_base_model/mechanical accessory loads <acc>/Mechanical Accessory Loads v2 <acc>/backward model/mechanical accessories (Nm)/Mechanical Accessories: Const Mech Var Elect/Elec Aux Loads 14V Pwr/HeatedSeats/Subsystem/Subsystem/DurationOn1 ==
  Constant : Constant  Value=DurationOn
  Out1 : Outport
  wires:
  Constant/1 -> Out1/1

== system BD_PAR_AUTO_base_model/mechanical accessory loads <acc>/Mechanical Accessory Loads v2 <acc>/backward model/mechanical accessories (Nm)/Mechanical Accessories: Const Mech Var Elect/Elec Aux Loads 14V Pwr/HeatedSeats/Subsystem/Subsystem/Period1 ==
  Constant : Constant  Value=Period
  Out1 : Outport
  wires:
  Constant/1 -> Out1/1

== system BD_PAR_AUTO_base_model/mechanical accessory loads <acc>/Mechanical Accessory Loads v2 <acc>/backward model/mechanical accessories (Nm)/Mechanical Accessories: Const Mech Var Elect/Elec Aux Loads 14V Pwr/HeatedSeats/Subsystem/Subsystem/StartTime1 ==
  Constant : Constant  Value=StartTime
  Out1 : Outport
  wires:
  Constant/1 -> Out1/1

== system BD_PAR_AUTO_base_model/mechanical accessory loads <acc>/Mechanical Accessory Loads v2 <acc>/backward model/mechanical accessories (Nm)/Mechanical Accessories: Const Mech Var Elect/Elec Aux Loads 14V Pwr/HeatedSeats/Subsystem/Subsystem/StartTime3 ==
  Constant : Constant  Value=StartTime
  Out1 : Outport
  wires:
  Constant/1 -> Out1/1

== system BD_PAR_AUTO_base_model/mechanical accessory loads <acc>/Mechanical Accessory Loads v2 <acc>/backward model/mechanical accessories (Nm)/Mechanical Accessories: Const Mech Var Elect/Elec Aux Loads 14V Pwr/HeatedSeats/Subsystem/Subsystem/Triggered Subsystem2 ==
  time : Inport
  Trigger : TriggerPort  VariantControl=(inherit)
  last trig on time : Outport  InitialOutput=StartTime
  wires:
  time/1 -> last trig on time/1

== system BD_PAR_AUTO_base_model/mechanical accessory loads <acc>/Mechanical Accessory Loads v2 <acc>/backward model/mechanical accessories (Nm)/Mechanical Accessories: Const Mech Var Elect/Elec Aux Loads 14V Pwr/HeatedSeats/Subsystem/Subsystem1/ToggleTimes ==
  Constant : Constant  Value=ToggleTimes  VectorParams1D=off
  Out1 : Outport
  wires:
  Constant/1 -> Out1/1

== system BD_PAR_AUTO_base_model/mechanical accessory loads <acc>/Mechanical Accessory Loads v2 <acc>/backward model/mechanical accessories (Nm)/Mechanical Accessories: Const Mech Var Elect/Elec Aux Loads 14V Pwr/HeatedSeats/Subsystem/Subsystem1/Triggered Subsystem1 ==
  In1 : Inport
  Enable : EnablePort
  Constant1 : Constant
  Constant2 : Constant  Value=0
  Constant3 : Constant  Value=0
  Relational Operator : RelationalOperator  Operator===  RndMeth=Nearest  InputSameDT=on
  Switch : Switch  Threshold=.5
  Out1 : Outport  InitialOutput=InitialOn
  wires:
  Switch/1 -> Out1/1
  Constant3/1 -> Switch/3
  Constant1/1 -> Switch/1
  Relational Operator/1 -> Switch/2
  Constant2/1 -> Relational Operator/2
  In1/1 -> Relational Operator/1

== system BD_PAR_AUTO_base_model/mechanical accessory loads <acc>/Mechanical Accessory Loads v2 <acc>/backward model/mechanical accessories (Nm)/Mechanical Accessories: Const Mech Var Elect/Elec Aux Loads 14V Pwr/RadiatorCoolingFan/Subsystem/Subsystem/DurationOn1 ==
  Constant : Constant  Value=DurationOn
  Out1 : Outport
  wires:
  Constant/1 -> Out1/1

== system BD_PAR_AUTO_base_model/mechanical accessory loads <acc>/Mechanical Accessory Loads v2 <acc>/backward model/mechanical accessories (Nm)/Mechanical Accessories: Const Mech Var Elect/Elec Aux Loads 14V Pwr/RadiatorCoolingFan/Subsystem/Subsystem/Period1 ==
  Constant : Constant  Value=Period
  Out1 : Outport
  wires:
  Constant/1 -> Out1/1

== system BD_PAR_AUTO_base_model/mechanical accessory loads <acc>/Mechanical Accessory Loads v2 <acc>/backward model/mechanical accessories (Nm)/Mechanical Accessories: Const Mech Var Elect/Elec Aux Loads 14V Pwr/RadiatorCoolingFan/Subsystem/Subsystem/StartTime1 ==
  Constant : Constant  Value=StartTime
  Out1 : Outport
  wires:
  Constant/1 -> Out1/1

== system BD_PAR_AUTO_base_model/mechanical accessory loads <acc>/Mechanical Accessory Loads v2 <acc>/backward model/mechanical accessories (Nm)/Mechanical Accessories: Const Mech Var Elect/Elec Aux Loads 14V Pwr/RadiatorCoolingFan/Subsystem/Subsystem/StartTime3 ==
  Constant : Constant  Value=StartTime
  Out1 : Outport
  wires:
  Constant/1 -> Out1/1

== system BD_PAR_AUTO_base_model/mechanical accessory loads <acc>/Mechanical Accessory Loads v2 <acc>/backward model/mechanical accessories (Nm)/Mechanical Accessories: Const Mech Var Elect/Elec Aux Loads 14V Pwr/RadiatorCoolingFan/Subsystem/Subsystem/Triggered Subsystem2 ==
  time : Inport
  Trigger : TriggerPort  VariantControl=(inherit)
  last trig on time : Outport  InitialOutput=StartTime
  wires:
  time/1 -> last trig on time/1

== system BD_PAR_AUTO_base_model/mechanical accessory loads <acc>/Mechanical Accessory Loads v2 <acc>/backward model/mechanical accessories (Nm)/Mechanical Accessories: Const Mech Var Elect/Elec Aux Loads 14V Pwr/RadiatorCoolingFan/Subsystem/Subsystem1/ToggleTimes ==
  Constant : Constant  Value=ToggleTimes  VectorParams1D=off
  Out1 : Outport
  wires:
  Constant/1 -> Out1/1

== system BD_PAR_AUTO_base_model/mechanical accessory loads <acc>/Mechanical Accessory Loads v2 <acc>/backward model/mechanical accessories (Nm)/Mechanical Accessories: Const Mech Var Elect/Elec Aux Loads 14V Pwr/RadiatorCoolingFan/Subsystem/Subsystem1/Triggered Subsystem1 ==
  In1 : Inport
  Enable : EnablePort
  Constant1 : Constant
  Constant2 : Constant  Value=0
  Constant3 : Constant  Value=0
  Relational Operator : RelationalOperator  Operator===  RndMeth=Nearest  InputSameDT=on
  Switch : Switch  Threshold=.5
  Out1 : Outport  InitialOutput=InitialOn
  wires:
  Switch/1 -> Out1/1
  Constant3/1 -> Switch/3
  Constant1/1 -> Switch/1
  Relational Operator/1 -> Switch/2
  Constant2/1 -> Relational Operator/2
  In1/1 -> Relational Operator/1

== system BD_PAR_AUTO_base_model/mechanical accessory loads <acc>/Mechanical Accessory Loads v2 <acc>/backward model/mechanical accessories (Nm)/Mechanical Accessories: Const Mech Var Elect/Elec Aux Loads 14V Pwr/Radio/Subsystem/Subsystem/DurationOn1 ==
  Constant : Constant  Value=DurationOn
  Out1 : Outport
  wires:
  Constant/1 -> Out1/1

== system BD_PAR_AUTO_base_model/mechanical accessory loads <acc>/Mechanical Accessory Loads v2 <acc>/backward model/mechanical accessories (Nm)/Mechanical Accessories: Const Mech Var Elect/Elec Aux Loads 14V Pwr/Radio/Subsystem/Subsystem/Period1 ==
  Constant : Constant  Value=Period
  Out1 : Outport
  wires:
  Constant/1 -> Out1/1

== system BD_PAR_AUTO_base_model/mechanical accessory loads <acc>/Mechanical Accessory Loads v2 <acc>/backward model/mechanical accessories (Nm)/Mechanical Accessories: Const Mech Var Elect/Elec Aux Loads 14V Pwr/Radio/Subsystem/Subsystem/StartTime1 ==
  Constant : Constant  Value=StartTime
  Out1 : Outport
  wires:
  Constant/1 -> Out1/1

== system BD_PAR_AUTO_base_model/mechanical accessory loads <acc>/Mechanical Accessory Loads v2 <acc>/backward model/mechanical accessories (Nm)/Mechanical Accessories: Const Mech Var Elect/Elec Aux Loads 14V Pwr/Radio/Subsystem/Subsystem/StartTime3 ==
  Constant : Constant  Value=StartTime
  Out1 : Outport
  wires:
  Constant/1 -> Out1/1

== system BD_PAR_AUTO_base_model/mechanical accessory loads <acc>/Mechanical Accessory Loads v2 <acc>/backward model/mechanical accessories (Nm)/Mechanical Accessories: Const Mech Var Elect/Elec Aux Loads 14V Pwr/Radio/Subsystem/Subsystem/Triggered Subsystem2 ==
  time : Inport
  Trigger : TriggerPort  VariantControl=(inherit)
  last trig on time : Outport  InitialOutput=StartTime
  wires:
  time/1 -> last trig on time/1

== system BD_PAR_AUTO_base_model/mechanical accessory loads <acc>/Mechanical Accessory Loads v2 <acc>/backward model/mechanical accessories (Nm)/Mechanical Accessories: Const Mech Var Elect/Elec Aux Loads 14V Pwr/Radio/Subsystem/Subsystem1/ToggleTimes ==
  Constant : Constant  Value=ToggleTimes  VectorParams1D=off
  Out1 : Outport
  wires:
  Constant/1 -> Out1/1

== system BD_PAR_AUTO_base_model/mechanical accessory loads <acc>/Mechanical Accessory Loads v2 <acc>/backward model/mechanical accessories (Nm)/Mechanical Accessories: Const Mech Var Elect/Elec Aux Loads 14V Pwr/Radio/Subsystem/Subsystem1/Triggered Subsystem1 ==
  In1 : Inport
  Enable : EnablePort
  Constant1 : Constant
  Constant2 : Constant  Value=0
  Constant3 : Constant  Value=0
  Relational Operator : RelationalOperator  Operator===  RndMeth=Nearest  InputSameDT=on
  Switch : Switch  Threshold=.5
  Out1 : Outport  InitialOutput=InitialOn
  wires:
  Switch/1 -> Out1/1
  Constant3/1 -> Switch/3
  Constant1/1 -> Switch/1
  Relational Operator/1 -> Switch/2
  Constant2/1 -> Relational Operator/2
  In1/1 -> Relational Operator/1

== system BD_PAR_AUTO_base_model/mechanical accessory loads <acc>/Mechanical Accessory Loads v2 <acc>/backward model/mechanical accessories (Nm)/Mechanical Accessories: Const Mech Var Elect/Elec Aux Loads 14V Pwr/RearDefrost/Subsystem/Subsystem/DurationOn1 ==
  Constant : Constant  Value=DurationOn
  Out1 : Outport
  wires:
  Constant/1 -> Out1/1

== system BD_PAR_AUTO_base_model/mechanical accessory loads <acc>/Mechanical Accessory Loads v2 <acc>/backward model/mechanical accessories (Nm)/Mechanical Accessories: Const Mech Var Elect/Elec Aux Loads 14V Pwr/RearDefrost/Subsystem/Subsystem/Period1 ==
  Constant : Constant  Value=Period
  Out1 : Outport
  wires:
  Constant/1 -> Out1/1

== system BD_PAR_AUTO_base_model/mechanical accessory loads <acc>/Mechanical Accessory Loads v2 <acc>/backward model/mechanical accessories (Nm)/Mechanical Accessories: Const Mech Var Elect/Elec Aux Loads 14V Pwr/RearDefrost/Subsystem/Subsystem/StartTime1 ==
  Constant : Constant  Value=StartTime
  Out1 : Outport
  wires:
  Constant/1 -> Out1/1

== system BD_PAR_AUTO_base_model/mechanical accessory loads <acc>/Mechanical Accessory Loads v2 <acc>/backward model/mechanical accessories (Nm)/Mechanical Accessories: Const Mech Var Elect/Elec Aux Loads 14V Pwr/RearDefrost/Subsystem/Subsystem/StartTime3 ==
  Constant : Constant  Value=StartTime
  Out1 : Outport
  wires:
  Constant/1 -> Out1/1

== system BD_PAR_AUTO_base_model/mechanical accessory loads <acc>/Mechanical Accessory Loads v2 <acc>/backward model/mechanical accessories (Nm)/Mechanical Accessories: Const Mech Var Elect/Elec Aux Loads 14V Pwr/RearDefrost/Subsystem/Subsystem/Triggered Subsystem2 ==
  time : Inport
  Trigger : TriggerPort  VariantControl=(inherit)
  last trig on time : Outport  InitialOutput=StartTime
  wires:
  time/1 -> last trig on time/1

== system BD_PAR_AUTO_base_model/mechanical accessory loads <acc>/Mechanical Accessory Loads v2 <acc>/backward model/mechanical accessories (Nm)/Mechanical Accessories: Const Mech Var Elect/Elec Aux Loads 14V Pwr/RearDefrost/Subsystem/Subsystem1/ToggleTimes ==
  Constant : Constant  Value=ToggleTimes  VectorParams1D=off
  Out1 : Outport
  wires:
  Constant/1 -> Out1/1

== system BD_PAR_AUTO_base_model/mechanical accessory loads <acc>/Mechanical Accessory Loads v2 <acc>/backward model/mechanical accessories (Nm)/Mechanical Accessories: Const Mech Var Elect/Elec Aux Loads 14V Pwr/RearDefrost/Subsystem/Subsystem1/Triggered Subsystem1 ==
  In1 : Inport
  Enable : EnablePort
  Constant1 : Constant
  Constant2 : Constant  Value=0
  Constant3 : Constant  Value=0
  Relational Operator : RelationalOperator  Operator===  RndMeth=Nearest  InputSameDT=on
  Switch : Switch  Threshold=.5
  Out1 : Outport  InitialOutput=InitialOn
  wires:
  Switch/1 -> Out1/1
  Constant3/1 -> Switch/3
  Constant1/1 -> Switch/1
  Relational Operator/1 -> Switch/2
  Constant2/1 -> Relational Operator/2
  In1/1 -> Relational Operator/1

== system BD_PAR_AUTO_base_model/mechanical accessory loads <acc>/Mechanical Accessory Loads v2 <acc>/backward model/mechanical accessories (Nm)/Mechanical Accessories: Const Mech Var Elect/Elec Aux Loads 14V Pwr/RearHVAC/Subsystem/Subsystem/DurationOn1 ==
  Constant : Constant  Value=DurationOn
  Out1 : Outport
  wires:
  Constant/1 -> Out1/1

== system BD_PAR_AUTO_base_model/mechanical accessory loads <acc>/Mechanical Accessory Loads v2 <acc>/backward model/mechanical accessories (Nm)/Mechanical Accessories: Const Mech Var Elect/Elec Aux Loads 14V Pwr/RearHVAC/Subsystem/Subsystem/Period1 ==
  Constant : Constant  Value=Period
  Out1 : Outport
  wires:
  Constant/1 -> Out1/1

== system BD_PAR_AUTO_base_model/mechanical accessory loads <acc>/Mechanical Accessory Loads v2 <acc>/backward model/mechanical accessories (Nm)/Mechanical Accessories: Const Mech Var Elect/Elec Aux Loads 14V Pwr/RearHVAC/Subsystem/Subsystem/StartTime1 ==
  Constant : Constant  Value=StartTime
  Out1 : Outport
  wires:
  Constant/1 -> Out1/1

== system BD_PAR_AUTO_base_model/mechanical accessory loads <acc>/Mechanical Accessory Loads v2 <acc>/backward model/mechanical accessories (Nm)/Mechanical Accessories: Const Mech Var Elect/Elec Aux Loads 14V Pwr/RearHVAC/Subsystem/Subsystem/StartTime3 ==
  Constant : Constant  Value=StartTime
  Out1 : Outport
  wires:
  Constant/1 -> Out1/1

== system BD_PAR_AUTO_base_model/mechanical accessory loads <acc>/Mechanical Accessory Loads v2 <acc>/backward model/mechanical accessories (Nm)/Mechanical Accessories: Const Mech Var Elect/Elec Aux Loads 14V Pwr/RearHVAC/Subsystem/Subsystem/Triggered Subsystem2 ==
  time : Inport
  Trigger : TriggerPort  VariantControl=(inherit)
  last trig on time : Outport  InitialOutput=StartTime
  wires:
  time/1 -> last trig on time/1

== system BD_PAR_AUTO_base_model/mechanical accessory loads <acc>/Mechanical Accessory Loads v2 <acc>/backward model/mechanical accessories (Nm)/Mechanical Accessories: Const Mech Var Elect/Elec Aux Loads 14V Pwr/RearHVAC/Subsystem/Subsystem1/ToggleTimes ==
  Constant : Constant  Value=ToggleTimes  VectorParams1D=off
  Out1 : Outport
  wires:
  Constant/1 -> Out1/1

== system BD_PAR_AUTO_base_model/mechanical accessory loads <acc>/Mechanical Accessory Loads v2 <acc>/backward model/mechanical accessories (Nm)/Mechanical Accessories: Const Mech Var Elect/Elec Aux Loads 14V Pwr/RearHVAC/Subsystem/Subsystem1/Triggered Subsystem1 ==
  In1 : Inport
  Enable : EnablePort
  Constant1 : Constant
  Constant2 : Constant  Value=0
  Constant3 : Constant  Value=0
  Relational Operator : RelationalOperator  Operator===  RndMeth=Nearest  InputSameDT=on
  Switch : Switch  Threshold=.5
  Out1 : Outport  InitialOutput=InitialOn
  wires:
  Switch/1 -> Out1/1
  Constant3/1 -> Switch/3
  Constant1/1 -> Switch/1
  Relational Operator/1 -> Switch/2
  Constant2/1 -> Relational Operator/2
  In1/1 -> Relational Operator/1

== system BD_PAR_AUTO_base_model/mechanical accessory loads <acc>/Mechanical Accessory Loads v2 <acc>/backward model/mechanical accessories (Nm)/Mechanical Accessories: Const Mech Var Elect/Elec Aux Loads 14V Pwr/RearWipers/Subsystem/Subsystem/DurationOn1 ==
  Constant : Constant  Value=DurationOn
  Out1 : Outport
  wires:
  Constant/1 -> Out1/1

== system BD_PAR_AUTO_base_model/mechanical accessory loads <acc>/Mechanical Accessory Loads v2 <acc>/backward model/mechanical accessories (Nm)/Mechanical Accessories: Const Mech Var Elect/Elec Aux Loads 14V Pwr/RearWipers/Subsystem/Subsystem/Period1 ==
  Constant : Constant  Value=Period
  Out1 : Outport
  wires:
  Constant/1 -> Out1/1

== system BD_PAR_AUTO_base_model/mechanical accessory loads <acc>/Mechanical Accessory Loads v2 <acc>/backward model/mechanical accessories (Nm)/Mechanical Accessories: Const Mech Var Elect/Elec Aux Loads 14V Pwr/RearWipers/Subsystem/Subsystem/StartTime1 ==
  Constant : Constant  Value=StartTime
  Out1 : Outport
  wires:
  Constant/1 -> Out1/1

== system BD_PAR_AUTO_base_model/mechanical accessory loads <acc>/Mechanical Accessory Loads v2 <acc>/backward model/mechanical accessories (Nm)/Mechanical Accessories: Const Mech Var Elect/Elec Aux Loads 14V Pwr/RearWipers/Subsystem/Subsystem/StartTime3 ==
  Constant : Constant  Value=StartTime
  Out1 : Outport
  wires:
  Constant/1 -> Out1/1

== system BD_PAR_AUTO_base_model/mechanical accessory loads <acc>/Mechanical Accessory Loads v2 <acc>/backward model/mechanical accessories (Nm)/Mechanical Accessories: Const Mech Var Elect/Elec Aux Loads 14V Pwr/RearWipers/Subsystem/Subsystem/Triggered Subsystem2 ==
  time : Inport
  Trigger : TriggerPort  VariantControl=(inherit)
  last trig on time : Outport  InitialOutput=StartTime
  wires:
  time/1 -> last trig on time/1

== system BD_PAR_AUTO_base_model/mechanical accessory loads <acc>/Mechanical Accessory Loads v2 <acc>/backward model/mechanical accessories (Nm)/Mechanical Accessories: Const Mech Var Elect/Elec Aux Loads 14V Pwr/RearWipers/Subsystem/Subsystem1/ToggleTimes ==
  Constant : Constant  Value=ToggleTimes  VectorParams1D=off
  Out1 : Outport
  wires:
  Constant/1 -> Out1/1

== system BD_PAR_AUTO_base_model/mechanical accessory loads <acc>/Mechanical Accessory Loads v2 <acc>/backward model/mechanical accessories (Nm)/Mechanical Accessories: Const Mech Var Elect/Elec Aux Loads 14V Pwr/RearWipers/Subsystem/Subsystem1/Triggered Subsystem1 ==
  In1 : Inport
  Enable : EnablePort
  Constant1 : Constant
  Constant2 : Constant  Value=0
  Constant3 : Constant  Value=0
  Relational Operator : RelationalOperator  Operator===  RndMeth=Nearest  InputSameDT=on
  Switch : Switch  Threshold=.5
  Out1 : Outport  InitialOutput=InitialOn
  wires:
  Switch/1 -> Out1/1
  Constant3/1 -> Switch/3
  Constant1/1 -> Switch/1
  Relational Operator/1 -> Switch/2
  Constant2/1 -> Relational Operator/2
  In1/1 -> Relational Operator/1

== system BD_PAR_AUTO_base_model/mechanical accessory loads <acc>/Mechanical Accessory Loads v2 <acc>/backward model/mechanical accessories (Nm)/Mechanical Accessories: Const Mech Var Elect/Elec Aux Loads 14V Pwr/Starter/Starter/Subsystem/Last Engine On Time ==
  In1 : Inport
  Trigger : TriggerPort  VariantControl=(inherit)
  Out1 : Outport  InitialOutput=-100
  wires:
  In1/1 -> Out1/1

== system BD_PAR_AUTO_base_model/mechanical accessory loads <acc>/Mechanical Accessory Loads v2 <acc>/backward model/mechanical accessories (Nm)/Mechanical Accessories: Const Mech Var Elect/Elec Aux Loads 14V Pwr/TurnSignals/Subsystem/Subsystem/DurationOn1 ==
  Constant : Constant  Value=DurationOn
  Out1 : Outport
  wires:
  Constant/1 -> Out1/1
